simulink model "matlab_serial"  (R2024b)
settings: Solver=VariableStepAuto  StartTime=0.0  StopTime=10.0  RelTol=1e-3
libraries: instrumentseriallib x3
settings Model: Creator=nl  LastModifiedBy=nl

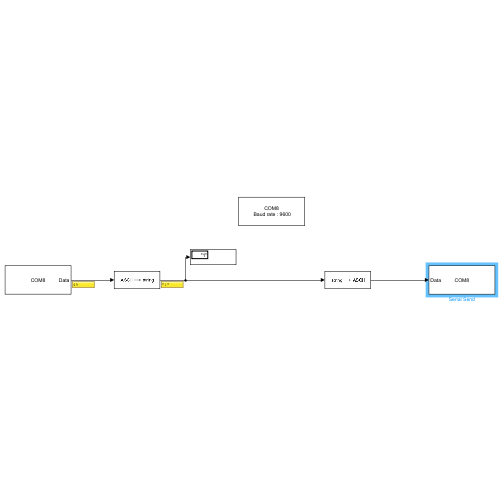
[thumbnail: Simulink's stored preview of the top-level diagram]
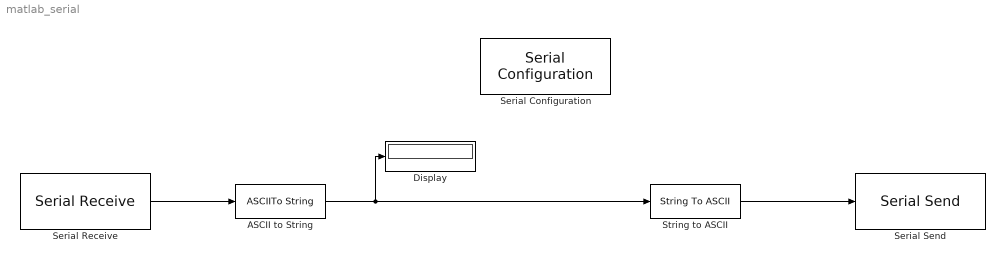
== system matlab_serial ==
  ASCII to String : ASCIIToString
  Display : Display
  Serial Configuration : instrumentseriallib/Serial Configuration  Priority=-200000  PortSel=COM8  Port=COM8  ComPort=COM8  BaudRate=9600  DataBits=8  Parity=none  StopBits=1  ByteOrder=little-endian  FlowControl=none  Timeout=10  SimulateUsing=Interpreted execution  BlockInModel=on  aMode=1
  Serial Receive : instrumentseriallib/Serial Receive  Priority=1  PortSel=COM8  Port=COM8  ComPort=COM8  DataType=uint8  SaveDataType=uint8  ToggleHeader=off  Header=['A']  ToggleDataSize=on  DataSize=[1]  ToggleTerminator=off  Terminator=Custom terminator  CustomTerminator=['#']  InputFormat=Column major  EnableBlockingMode=on  ActionDataUnavailable=Output last received value  ActionWhenDataUnavailable=Output last received value  CustomValue=0  SampleTime=0.01  SimulateUsing=Interpreted execution  BlockInModel=on  aMode=1
  Serial Send : instrumentseriallib/Serial Send  Priority=1  PortSel=COM8  Port=COM8  ComPort=COM8  Header=[]  Terminator=<none>  CustomTerminator=[]  EnableBlockingMode=on  SimulateUsing=Interpreted execution  BlockInModel=on  aMode=1
  String to ASCII : StringToASCII
  wires:
  Serial Receive/1 -> ASCII to String/1
  ASCII to String/1 -> String to ASCII/1, Display/1
  String to ASCII/1 -> Serial Send/1
